simulink library "InterModuleProtocol"  (R2023b)
settings: Solver=VariableStepAuto  StartTime=0.0  StopTime=10.0  RelTol=1e-3
undefined symbols (not defined in the file or in its folder): accelerationNED, accelerationNEDXYZ, accelerationXYZ, angleOfAttack, courseOverGround, orientationQuaternion, orientationRollPitchYaw, positionLLA, positionNED, sideSlipAngle, speedOverGround, velocityNED, velocityNEDUVW, velocityPQR, velocityUVW
libraries: $bdroot x10
(part 3 of 3)

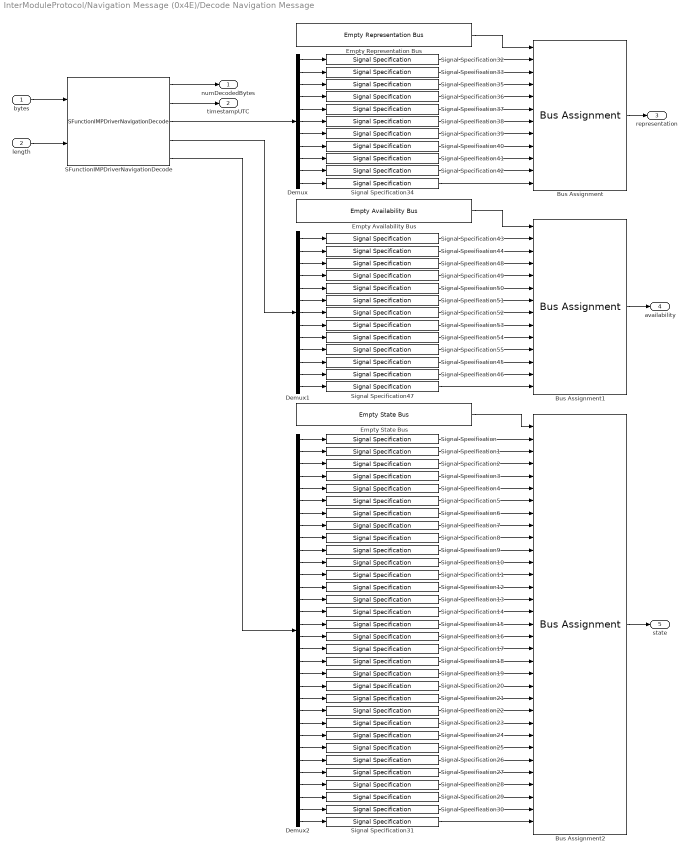
== system InterModuleProtocol/Navigation Message (0x4E)/Decode Navigation Message ==
  bytes : Inport  OutDataTypeStr=uint8
  length : Inport  Port=2  OutDataTypeStr=uint32  PortDimensions=1
  Bus Assignment : BusAssignment  AssignedSignals=positionLLA,positionNED,orientationQuaternion,orientationRollPitchYaw,velocityNEDUVW,velocityPQR,accelerationNEDXYZ,courseOverGround,speedOverGround,angleOfAttack,sideSlipAngle
  Bus Assignment1 : BusAssignment  AssignedSignals=positionLLA,positionNED,orientationQuaternion,orientationRollPitchYaw,velocityNED,velocityUVW,velocityPQR,accelerationNED,accelerationXYZ,courseOverGround,speedOverGround,angleOfAttack,sideSlipAngle
  Bus Assignment2 : BusAssignment  AssignedSignals=positionLatitude,positionLongitude,positionAltitude,positionNorth,positionEast,positionDown,orientationQuaternionW,orientationQuaternionX,orientationQuaternionY,orientationQuaternionZ,orientationRoll,orientationPitch,orientationYaw,velocityNorth,velocityEast,velocityDown,velocityU,velocityV,velocityW,velocityP,velocityQ,velocityR,accelerationNorth,accelerationEast,accelerationDown,accelerationX,accelerationY,accelerationZ,courseOverGround,speedOverGround,angleOfAttack,sideSlipAngle
  Demux : Demux  Outputs=11
  Demux1 : Demux  Outputs=13
  Demux2 : Demux  Outputs=32
  Empty Availability Bus : $bdroot/Empty Availability Bus
  Empty Representation Bus : $bdroot/Empty Representation Bus
  Empty State Bus : $bdroot/Empty State Bus
  SFunctionIMPDriverNavigationDecode : S-Function  FunctionName=SFunctionIMPDriverNavigationDecode  Parameters=SampleTime  SFunctionDeploymentMode=off  EnableBusSupport=off  mask(Legacy Function){SFunctionSpec=void IMP_OutputDriverNavigationDecode(uint8 u1[], uint32 u2, int32 y1[1], double y2[1], uint8 y3[11], uint8 y4[13], double y5[32]), SampleTime=-1, ShowSpec=off}
      mask prompts: SampleTime "Sample time (-1 for inherited):"; ShowSpec "Display function specification"
      mask help:
      | This block allows you to call the legacy functions specified by the following Legacy Code Tool definition:
      | def.SFunctionName = 'SFunctionIMPDriverNavigationDecode';
      | def.OutputFcnSpec = 'void IMP_OutputDriverNavigationDecode(uint8 u1[], uint32 u2, int32 y1[1], double y2[1], uint8 y3[11], uint8 y4[13], double y5[32])';
      | def.StartFcnSpec = 'void IMP_CreateDriverNavigationDecode()';
      | def.TerminateFcnSpec = 'void IMP_DeleteDriverNavigationDecode()';
      | def.HeaderFiles = {'IMP_DriverNavigationDecode.h'};
      | def.SourceFiles = {'IMP_DriverNavigationDecode.cpp', 'InterModuleProtocol.cpp', 'IMPConvexPolygon.cpp', 'IMPState.cpp', 'IMPStateConfiguration.cpp'};
      | def.IncPaths = {'..\..\source\InterModuleProtocol'};
      | def.SrcPaths = {'..\..\source\InterModuleProtocol'};
      | def.SampleTime = 'parameterized';
      | def.Options.useTlcWithAccel = false;
      mask Help: <p>This block was generated automatically by the Legacy Code Tool. For detailed help on this tool, call<a href="matlab:legacy_code('help')"> legacy_code('help')</a>.</p>
      mask Callback ShowSpec:
      | if strcmp(get_param(gcbh, 'ShowSpec'), 'on')
      |   set_param(gcbh, 'MaskDisplay', sprintf('fprintf(''%s'');', get_param(gcbh, 'SFunctionSpec')));
      | else
      |   set_param(gcbh, 'MaskDisplay', sprintf('fprintf(''%s'');', get_param(gcbh, 'FunctionName')));
      | end
      mask Display: fprintf('SFunctionIMPDriverNavigationDecode');
  Signal Specification{,1,10..12,28,30..31} (8 alike) : SignalSpecification  OutDataTypeStr=double  Unit=rad  Dimensions=1
  Signal Specification{13..18,29} (7 alike) : SignalSpecification  OutDataTypeStr=double  Unit=m/s  Dimensions=1
  Signal Specification19 : SignalSpecification  OutDataTypeStr=double  Unit=rad/s  Dimensions=1
  Signal Specification{2..5} (4 alike) : SignalSpecification  OutDataTypeStr=double  Unit=m  Dimensions=1
  Signal Specification20 : SignalSpecification  OutDataTypeStr=double  Unit=rad/s  Dimensions=1
  Signal Specification21 : SignalSpecification  OutDataTypeStr=double  Unit=rad/s  Dimensions=1
  Signal Specification{22..27} (6 alike) : SignalSpecification  OutDataTypeStr=double  Unit=m/s^2  Dimensions=1
  Signal Specification{32..55} (24 alike) : SignalSpecification  OutDataTypeStr=uint8  Dimensions=1
  Signal Specification{6..9} (4 alike) : SignalSpecification  OutDataTypeStr=double  Dimensions=1
  numDecodedBytes : Outport  OutDataTypeStr=int32  PortDimensions=1  VectorParamsAs1DForOutWhenUnconnected=off
  timestampUTC : Outport  Port=2  OutDataTypeStr=double  Unit=s  PortDimensions=1  VectorParamsAs1DForOutWhenUnconnected=off
  representation : Outport  Port=3  VectorParamsAs1DForOutWhenUnconnected=off
  availability : Outport  Port=4  VectorParamsAs1DForOutWhenUnconnected=off
  state : Outport  Port=5  VectorParamsAs1DForOutWhenUnconnected=off
  wires:
  SFunctionIMPDriverNavigationDecode/1 -> numDecodedBytes/1
  SFunctionIMPDriverNavigationDecode/2 -> timestampUTC/1
  length/1 -> SFunctionIMPDriverNavigationDecode/2
  bytes/1 -> SFunctionIMPDriverNavigationDecode/1
  Signal Specification32/1 -> Bus Assignment/2
  Signal Specification34/1 -> Bus Assignment/12
  Signal Specification39/1 -> Bus Assignment/8
  Signal Specification40/1 -> Bus Assignment/9
  Signal Specification41/1 -> Bus Assignment/10
  Signal Specification37/1 -> Bus Assignment/6
  Signal Specification36/1 -> Bus Assignment/5
  Signal Specification33/1 -> Bus Assignment/3
  Signal Specification35/1 -> Bus Assignment/4
  Signal Specification47/1 -> Bus Assignment1/14
  Signal Specification46/1 -> Bus Assignment1/13
  Signal Specification54/1 -> Bus Assignment1/10
  Signal Specification45/1 -> Bus Assignment1/12
  Signal Specification53/1 -> Bus Assignment1/9
  Signal Specification51/1 -> Bus Assignment1/7
  Signal Specification50/1 -> Bus Assignment1/6
  Signal Specification52/1 -> Bus Assignment1/8
  Signal Specification48/1 -> Bus Assignment1/4
  Demux1/10 -> Signal Specification55/1
  Signal Specification43/1 -> Bus Assignment1/2
  Bus Assignment1/1 -> availability/1
  Demux/3 -> Signal Specification35/1
  Demux/10 -> Signal Specification42/1
  Demux/7 -> Signal Specification39/1
  Demux/4 -> Signal Specification36/1
  SFunctionIMPDriverNavigationDecode/4 -> Demux1/1
  SFunctionIMPDriverNavigationDecode/3 -> Demux/1
  Demux2/26 -> Signal Specification25/1
  Demux2/9 -> Signal Specification8/1
  Demux2/3 -> Signal Specification2/1
  Demux2/24 -> Signal Specification23/1
  Demux2/5 -> Signal Specification4/1
  Demux2/25 -> Signal Specification24/1
  Signal Specification55/1 -> Bus Assignment1/11
  Demux2/30 -> Signal Specification29/1
  Demux2/18 -> Signal Specification17/1
  Demux2/22 -> Signal Specification21/1
  Signal Specification2/1 -> Bus Assignment2/4
  Signal Specification29/1 -> Bus Assignment2/31
  Signal Specification/1 -> Bus Assignment2/2
  Signal Specification27/1 -> Bus Assignment2/29
  Signal Specification26/1 -> Bus Assignment2/28
  Signal Specification42/1 -> Bus Assignment/11
  Signal Specification25/1 -> Bus Assignment2/27
  Signal Specification44/1 -> Bus Assignment1/3
  Signal Specification24/1 -> Bus Assignment2/26
  Signal Specification31/1 -> Bus Assignment2/33
  Signal Specification23/1 -> Bus Assignment2/25
  Signal Specification22/1 -> Bus Assignment2/24
  Signal Specification17/1 -> Bus Assignment2/19
  Signal Specification14/1 -> Bus Assignment2/16
  Signal Specification15/1 -> Bus Assignment2/17
  Signal Specification16/1 -> Bus Assignment2/18
  Signal Specification21/1 -> Bus Assignment2/23
  Signal Specification10/1 -> Bus Assignment2/12
  Signal Specification30/1 -> Bus Assignment2/32
  Signal Specification4/1 -> Bus Assignment2/6
  Signal Specification6/1 -> Bus Assignment2/8
  Demux/11 -> Signal Specification34/1
  Signal Specification9/1 -> Bus Assignment2/11
  Demux/6 -> Signal Specification38/1
  Signal Specification13/1 -> Bus Assignment2/15
  Demux/8 -> Signal Specification40/1
  Bus Assignment2/1 -> state/1
  Signal Specification8/1 -> Bus Assignment2/10
  Demux1/6 -> Signal Specification51/1
  Demux1/7 -> Signal Specification52/1
  Signal Specification20/1 -> Bus Assignment2/22
  Demux1/4 -> Signal Specification49/1
  Demux1/2 -> Signal Specification44/1
  Demux1/13 -> Signal Specification47/1
  Empty Availability Bus/1 -> Bus Assignment1/1
  Signal Specification3/1 -> Bus Assignment2/5
  Demux/1 -> Signal Specification32/1
  Demux1/3 -> Signal Specification48/1
  Signal Specification12/1 -> Bus Assignment2/14
  Demux1/5 -> Signal Specification50/1
  Demux/9 -> Signal Specification41/1
  Demux1/8 -> Signal Specification53/1
  Demux2/21 -> Signal Specification20/1
  Demux2/10 -> Signal Specification9/1
  Demux1/1 -> Signal Specification43/1
  Signal Specification1/1 -> Bus Assignment2/3
  Demux2/31 -> Signal Specification30/1
  Demux2/15 -> Signal Specification14/1
  Demux2/29 -> Signal Specification28/1
  Demux/2 -> Signal Specification33/1
  Demux1/12 -> Signal Specification46/1
  Demux2/23 -> Signal Specification22/1
  Demux2/4 -> Signal Specification3/1
  Signal Specification38/1 -> Bus Assignment/7
  Demux2/8 -> Signal Specification7/1
  Empty Representation Bus/1 -> Bus Assignment/1
  Demux2/1 -> Signal Specification/1
  Signal Specification18/1 -> Bus Assignment2/20
  Demux2/11 -> Signal Specification10/1
  Demux2/6 -> Signal Specification5/1
  Demux2/19 -> Signal Specification18/1
  Signal Specification5/1 -> Bus Assignment2/7
  Demux2/7 -> Signal Specification6/1
  Demux2/17 -> Signal Specification16/1
  Demux2/2 -> Signal Specification1/1
  Signal Specification11/1 -> Bus Assignment2/13
  Demux2/16 -> Signal Specification15/1
  Demux2/27 -> Signal Specification26/1
  Demux2/28 -> Signal Specification27/1
  Demux2/32 -> Signal Specification31/1
  Demux2/20 -> Signal Specification19/1
  Demux2/14 -> Signal Specification13/1
  Demux2/12 -> Signal Specification11/1
  Demux2/13 -> Signal Specification12/1
  Demux1/9 -> Signal Specification54/1
  Signal Specification28/1 -> Bus Assignment2/30
  SFunctionIMPDriverNavigationDecode/5 -> Demux2/1
  Demux1/11 -> Signal Specification45/1
  Empty State Bus/1 -> Bus Assignment2/1
  Bus Assignment/1 -> representation/1
  Signal Specification49/1 -> Bus Assignment1/5
  Demux/5 -> Signal Specification37/1
  Signal Specification7/1 -> Bus Assignment2/9
  Signal Specification19/1 -> Bus Assignment2/21

== system InterModuleProtocol/Navigation Message (0x4E)/Encode Navigation Message ==
  timestampUTC : Inport  OutDataTypeStr=double  Unit=s  PortDimensions=1
  representation : Inport  Port=2
  availability : Inport  Port=3
  state : Inport  Port=4
  Bus Selector : BusSelector  OutputSignals=positionLLA,positionNED,orientationQuaternion,orientationRollPitchYaw,velocityNEDUVW,velocityPQR,accelerationNEDXYZ,courseOverGround,speedOverGround,angleOfAttack,sideSlipAngle  OutputAsBus=on
  Bus Selector1 : BusSelector  OutputSignals=positionLLA,positionNED,orientationQuaternion,orientationRollPitchYaw,velocityNED,velocityUVW,velocityPQR,accelerationNED,accelerationXYZ,courseOverGround,speedOverGround,angleOfAttack,sideSlipAngle  OutputAsBus=on
  Bus Selector2 : BusSelector  OutputSignals=positionLatitude,positionLongitude,positionAltitude,positionNorth,positionEast,positionDown,orientationQuaternionW,orientationQuaternionX,orientationQuaternionY,orientationQuaternionZ,orientationRoll,orientationPitch,orientationYaw,velocityNorth,velocityEast,velocityDown,velocityU,velocityV,velocityW,velocityP,velocityQ,velocityR,accelerationNorth,accelerationEast,accelerationDown,accelerationX,accelerationY,accelerationZ,courseOverGround,speedOverGround,angleOfAttack,sideSlipAngle  OutputAsBus=on
  Bus to Vector : BusToVector
  Bus to Vector1 : BusToVector
  Bus to Vector2 : BusToVector
  Data Type Conversion : DataTypeConversion  OutDataTypeStr=uint8  SaturateOnIntegerOverflow=off  RndMeth=Floor
  Data Type Conversion1 : DataTypeConversion  OutDataTypeStr=uint8  SaturateOnIntegerOverflow=off  RndMeth=Floor
  Data Type Conversion2 : DataTypeConversion  OutDataTypeStr=double  SaturateOnIntegerOverflow=off  RndMeth=Floor
  SFunctionIMPDriverNavigationEncode : S-Function  FunctionName=SFunctionIMPDriverNavigationEncode  Parameters=SParameter1, SampleTime  SFunctionDeploymentMode=off  EnableBusSupport=off  mask(Legacy Function){SFunctionSpec=void IMP_OutputDriverNavigationEncode(uint8 y1[p1], uint32 y2[1], uint32 p1, double u1, uint8 u2[11], uint8 u3[13], double u4[32]), SParameter1=uint32(reshape(outputBufferSize, [1 1])), SampleTime=-1, ShowSpec=off}
      mask prompts: SParameter1 "P1:"; SampleTime "Sample time (-1 for inherited):"; ShowSpec "Display function specification"
      mask help:
      | This block allows you to call the legacy functions specified by the following Legacy Code Tool definition:
      | def.SFunctionName = 'SFunctionIMPDriverNavigationEncode';
      | def.OutputFcnSpec = 'void IMP_OutputDriverNavigationEncode(uint8 y1[p1], uint32 y2[1], uint32 p1, double u1, uint8 u2[11], uint8 u3[13], double u4[32])';
      | def.StartFcnSpec = 'void IMP_CreateDriverNavigationEncode()';
      | def.TerminateFcnSpec = 'void IMP_DeleteDriverNavigationEncode()';
      | def.HeaderFiles = {'IMP_DriverNavigationEncode.h'};
      | def.SourceFiles = {'IMP_DriverNavigationEncode.cpp', 'InterModuleProtocol.cpp', 'IMPConvexPolygon.cpp', 'IMPState.cpp', 'IMPStateConfiguration.cpp'};
      | def.IncPaths = {'..\..\source\InterModuleProtocol'};
      | def.SrcPaths = {'..\..\source\InterModuleProtocol'};
      | def.SampleTime = 'parameterized';
      | def.Options.useTlcWithAccel = false;
      mask Help: <p>This block was generated automatically by the Legacy Code Tool. For detailed help on this tool, call<a href="matlab:legacy_code('help')"> legacy_code('help')</a>.</p>
      mask Callback ShowSpec:
      | if strcmp(get_param(gcbh, 'ShowSpec'), 'on')
      |   set_param(gcbh, 'MaskDisplay', sprintf('fprintf(''%s'');', get_param(gcbh, 'SFunctionSpec')));
      | else
      |   set_param(gcbh, 'MaskDisplay', sprintf('fprintf(''%s'');', get_param(gcbh, 'FunctionName')));
      | end
      mask Display: fprintf('SFunctionIMPDriverNavigationEncode');
  bytes : Outport  OutDataTypeStr=uint8  PortDimensions=outputBufferSize  VectorParamsAs1DForOutWhenUnconnected=off
  length : Outport  Port=2  OutDataTypeStr=uint32  PortDimensions=1  VectorParamsAs1DForOutWhenUnconnected=off
  wires:
  SFunctionIMPDriverNavigationEncode/1 -> bytes/1
  timestampUTC/1 -> SFunctionIMPDriverNavigationEncode/1
  SFunctionIMPDriverNavigationEncode/2 -> length/1
  representation/1 -> Bus Selector/1
  Bus Selector/1 -> Bus to Vector/1
  state/1 -> Bus Selector2/1
  Data Type Conversion1/1 -> SFunctionIMPDriverNavigationEncode/3
  Data Type Conversion2/1 -> SFunctionIMPDriverNavigationEncode/4
  Bus to Vector1/1 -> Data Type Conversion1/1
  Data Type Conversion/1 -> SFunctionIMPDriverNavigationEncode/2
  availability/1 -> Bus Selector1/1
  Bus to Vector2/1 -> Data Type Conversion2/1
  Bus Selector2/1 -> Bus to Vector2/1
  Bus to Vector/1 -> Data Type Conversion/1
  Bus Selector1/1 -> Bus to Vector1/1
